simulink model "DriveSystemControl"  (R2025b)
settings: Solver=FixedStepAuto  StartTime=0.0  StopTime=Inf  FixedStep=0.001  RelTol=1e-3
PostLoadFcn:
  | if any(exist('dsrtsu_mdlpostloadfcn', 'file') ~= 0), dsrtsu_mdlpostloadfcn('Execute', bdroot); end
InitFcn:
  | , if any(exist('rtifpga_mdlclblib', 'file') ~= 0), rtifpga_mdlclblib('Init', bdroot); end,
  | , if any(exist('dsmpb_private', 'file') ~= 0), dsmpb_private('dsmpb_mdlclblib', 'Init', bdroot); end,
libraries: dsmpblib x2
(part 8 of 11)

== system DriveSystemControl/Bus Configuration (1) - In/Manipulation/gitam Controller CAN File 08082024/WIP/CANChannel/PDUs/TCU03/sigSupervisorFault/Feature Switch ==
  Const_sigSupervisorFault Countdown Start Value : Constant  Value=0  OutDataTypeStr=uint32
  Const_sigSupervisorFault Feature Switch : Constant  Value=0  OutDataTypeStr=uint32
  _Feature Switch_ : BusCreator  Inputs=2
  Feature Switch : Outport
  wires:
  _Feature Switch_/1 -> Feature Switch/1  "Feature Switch"
  Const_sigSupervisorFault Countdown Start Value/1 -> _Feature Switch_/1  "sigSupervisorFault Countdown Start Value"
  Const_sigSupervisorFault Feature Switch/1 -> _Feature Switch_/2  "sigSupervisorFault Feature Switch"

== system DriveSystemControl/Bus Configuration (1) - In/Manipulation/gitam Controller CAN File 08082024/WIP/CANChannel/PDUs/TCU03/sigSupervisorFault/ISignal Overwrite Value ==
  Const_sigSupervisorFault Overwrite Value : Constant  Value=0  OutDataTypeStr=uint8
  _ISignal Overwrite Value_ : BusCreator  Inputs=1
  ISignal Overwrite Value : Outport
  wires:
  _ISignal Overwrite Value_/1 -> ISignal Overwrite Value/1  "ISignal Overwrite Value"
  Const_sigSupervisorFault Overwrite Value/1 -> _ISignal Overwrite Value_/1  "sigSupervisorFault Overwrite Value"

== system DriveSystemControl/Bus Configuration (1) - In/Manipulation/gitam Controller CAN File 08082024/WIP/CANChannel/PDUs/TCU03/sigThrottlewiperHigh/Feature Switch ==
  Const_sigThrottlewiperHigh Countdown Start Value : Constant  Value=0  OutDataTypeStr=uint32
  Const_sigThrottlewiperHigh Feature Switch : Constant  Value=0  OutDataTypeStr=uint32
  _Feature Switch_ : BusCreator  Inputs=2
  Feature Switch : Outport
  wires:
  _Feature Switch_/1 -> Feature Switch/1  "Feature Switch"
  Const_sigThrottlewiperHigh Countdown Start Value/1 -> _Feature Switch_/1  "sigThrottlewiperHigh Countdown Start Value"
  Const_sigThrottlewiperHigh Feature Switch/1 -> _Feature Switch_/2  "sigThrottlewiperHigh Feature Switch"

== system DriveSystemControl/Bus Configuration (1) - In/Manipulation/gitam Controller CAN File 08082024/WIP/CANChannel/PDUs/TCU03/sigThrottlewiperHigh/ISignal Overwrite Value ==
  Const_sigThrottlewiperHigh Overwrite Value : Constant  Value=0  OutDataTypeStr=uint8
  _ISignal Overwrite Value_ : BusCreator  Inputs=1
  ISignal Overwrite Value : Outport
  wires:
  _ISignal Overwrite Value_/1 -> ISignal Overwrite Value/1  "ISignal Overwrite Value"
  Const_sigThrottlewiperHigh Overwrite Value/1 -> _ISignal Overwrite Value_/1  "sigThrottlewiperHigh Overwrite Value"

== system DriveSystemControl/Bus Configuration (1) - In/Manipulation/gitam Controller CAN File 08082024/WIP/CANChannel/PDUs/TCU03/sigThrottlewiperLow/Feature Switch ==
  Const_sigThrottlewiperLow Countdown Start Value : Constant  Value=0  OutDataTypeStr=uint32
  Const_sigThrottlewiperLow Feature Switch : Constant  Value=0  OutDataTypeStr=uint32
  _Feature Switch_ : BusCreator  Inputs=2
  Feature Switch : Outport
  wires:
  _Feature Switch_/1 -> Feature Switch/1  "Feature Switch"
  Const_sigThrottlewiperLow Countdown Start Value/1 -> _Feature Switch_/1  "sigThrottlewiperLow Countdown Start Value"
  Const_sigThrottlewiperLow Feature Switch/1 -> _Feature Switch_/2  "sigThrottlewiperLow Feature Switch"

== system DriveSystemControl/Bus Configuration (1) - In/Manipulation/gitam Controller CAN File 08082024/WIP/CANChannel/PDUs/TCU03/sigThrottlewiperLow/ISignal Overwrite Value ==
  Const_sigThrottlewiperLow Overwrite Value : Constant  Value=0  OutDataTypeStr=uint8
  _ISignal Overwrite Value_ : BusCreator  Inputs=1
  ISignal Overwrite Value : Outport
  wires:
  _ISignal Overwrite Value_/1 -> ISignal Overwrite Value/1  "ISignal Overwrite Value"
  Const_sigThrottlewiperLow Overwrite Value/1 -> _ISignal Overwrite Value_/1  "sigThrottlewiperLow Overwrite Value"

== system DriveSystemControl/Bus Configuration (1) - In/Manipulation/gitam Controller CAN File 08082024/WIP/CANChannel/PDUs/TCU03/sigVCLRunTimeError/Feature Switch ==
  Const_sigVCLRunTimeError Countdown Start Value : Constant  Value=0  OutDataTypeStr=uint32
  Const_sigVCLRunTimeError Feature Switch : Constant  Value=0  OutDataTypeStr=uint32
  _Feature Switch_ : BusCreator  Inputs=2
  Feature Switch : Outport
  wires:
  _Feature Switch_/1 -> Feature Switch/1  "Feature Switch"
  Const_sigVCLRunTimeError Countdown Start Value/1 -> _Feature Switch_/1  "sigVCLRunTimeError Countdown Start Value"
  Const_sigVCLRunTimeError Feature Switch/1 -> _Feature Switch_/2  "sigVCLRunTimeError Feature Switch"

== system DriveSystemControl/Bus Configuration (1) - In/Manipulation/gitam Controller CAN File 08082024/WIP/CANChannel/PDUs/TCU03/sigVCLRunTimeError/ISignal Overwrite Value ==
  Const_sigVCLRunTimeError Overwrite Value : Constant  Value=0  OutDataTypeStr=uint8
  _ISignal Overwrite Value_ : BusCreator  Inputs=1
  ISignal Overwrite Value : Outport
  wires:
  _ISignal Overwrite Value_/1 -> ISignal Overwrite Value/1  "ISignal Overwrite Value"
  Const_sigVCLRunTimeError Overwrite Value/1 -> _ISignal Overwrite Value_/1  "sigVCLRunTimeError Overwrite Value"

== system DriveSystemControl/Bus Configuration (1) - In/Manipulation/gitam Controller CAN File 08082024/WIP/CANChannel/PDUs/TCU04/sigMCU5_DriveMode/Feature Switch ==
  Const_sigMCU5_DriveMode Countdown Start Value : Constant  Value=0  OutDataTypeStr=uint32
  Const_sigMCU5_DriveMode Feature Switch : Constant  Value=0  OutDataTypeStr=uint32
  _Feature Switch_ : BusCreator  Inputs=2
  Feature Switch : Outport
  wires:
  _Feature Switch_/1 -> Feature Switch/1  "Feature Switch"
  Const_sigMCU5_DriveMode Countdown Start Value/1 -> _Feature Switch_/1  "sigMCU5_DriveMode Countdown Start Value"
  Const_sigMCU5_DriveMode Feature Switch/1 -> _Feature Switch_/2  "sigMCU5_DriveMode Feature Switch"

== system DriveSystemControl/Bus Configuration (1) - In/Manipulation/gitam Controller CAN File 08082024/WIP/CANChannel/PDUs/TCU04/sigMCU5_DriveMode/ISignal Overwrite Value ==
  Const_sigMCU5_DriveMode Overwrite Value : Constant  Value=0  OutDataTypeStr=uint8
  _ISignal Overwrite Value_ : BusCreator  Inputs=1
  ISignal Overwrite Value : Outport
  wires:
  _ISignal Overwrite Value_/1 -> ISignal Overwrite Value/1  "ISignal Overwrite Value"
  Const_sigMCU5_DriveMode Overwrite Value/1 -> _ISignal Overwrite Value_/1  "sigMCU5_DriveMode Overwrite Value"

== system DriveSystemControl/Bus Configuration (1) - In/Manipulation/gitam Controller CAN File 08082024/WIP/CANChannel/PDUs/TCU04/sigMCU5_Efficiency/Feature Switch ==
  Const_sigMCU5_Efficiency Countdown Start Value : Constant  Value=0  OutDataTypeStr=uint32
  Const_sigMCU5_Efficiency Feature Switch : Constant  Value=0  OutDataTypeStr=uint32
  _Feature Switch_ : BusCreator  Inputs=2
  Feature Switch : Outport
  wires:
  _Feature Switch_/1 -> Feature Switch/1  "Feature Switch"
  Const_sigMCU5_Efficiency Countdown Start Value/1 -> _Feature Switch_/1  "sigMCU5_Efficiency Countdown Start Value"
  Const_sigMCU5_Efficiency Feature Switch/1 -> _Feature Switch_/2  "sigMCU5_Efficiency Feature Switch"

== system DriveSystemControl/Bus Configuration (1) - In/Manipulation/gitam Controller CAN File 08082024/WIP/CANChannel/PDUs/TCU04/sigMCU5_Efficiency/ISignal Overwrite Value ==
  Const_sigMCU5_Efficiency Overwrite Value : Constant  Value=0  OutDataTypeStr=uint8
  _ISignal Overwrite Value_ : BusCreator  Inputs=1
  ISignal Overwrite Value : Outport
  wires:
  _ISignal Overwrite Value_/1 -> ISignal Overwrite Value/1  "ISignal Overwrite Value"
  Const_sigMCU5_Efficiency Overwrite Value/1 -> _ISignal Overwrite Value_/1  "sigMCU5_Efficiency Overwrite Value"

== system DriveSystemControl/Bus Configuration (1) - In/Manipulation/gitam Controller CAN File 08082024/WIP/CANChannel/PDUs/TCU04/sigMCU5_Hillhold/Feature Switch ==
  Const_sigMCU5_Hillhold Countdown Start Value : Constant  Value=0  OutDataTypeStr=uint32
  Const_sigMCU5_Hillhold Feature Switch : Constant  Value=0  OutDataTypeStr=uint32
  _Feature Switch_ : BusCreator  Inputs=2
  Feature Switch : Outport
  wires:
  _Feature Switch_/1 -> Feature Switch/1  "Feature Switch"
  Const_sigMCU5_Hillhold Countdown Start Value/1 -> _Feature Switch_/1  "sigMCU5_Hillhold Countdown Start Value"
  Const_sigMCU5_Hillhold Feature Switch/1 -> _Feature Switch_/2  "sigMCU5_Hillhold Feature Switch"

== system DriveSystemControl/Bus Configuration (1) - In/Manipulation/gitam Controller CAN File 08082024/WIP/CANChannel/PDUs/TCU04/sigMCU5_Hillhold/ISignal Overwrite Value ==
  Const_sigMCU5_Hillhold Overwrite Value : Constant  Value=0  OutDataTypeStr=uint8
  _ISignal Overwrite Value_ : BusCreator  Inputs=1
  ISignal Overwrite Value : Outport
  wires:
  _ISignal Overwrite Value_/1 -> ISignal Overwrite Value/1  "ISignal Overwrite Value"
  Const_sigMCU5_Hillhold Overwrite Value/1 -> _ISignal Overwrite Value_/1  "sigMCU5_Hillhold Overwrite Value"

== system DriveSystemControl/Bus Configuration (1) - In/Manipulation/gitam Controller CAN File 08082024/WIP/CANChannel/PDUs/TCU04/sigMCU5_RegenFlag/Feature Switch ==
  Const_sigMCU5_RegenFlag Countdown Start Value : Constant  Value=0  OutDataTypeStr=uint32
  Const_sigMCU5_RegenFlag Feature Switch : Constant  Value=0  OutDataTypeStr=uint32
  _Feature Switch_ : BusCreator  Inputs=2
  Feature Switch : Outport
  wires:
  _Feature Switch_/1 -> Feature Switch/1  "Feature Switch"
  Const_sigMCU5_RegenFlag Countdown Start Value/1 -> _Feature Switch_/1  "sigMCU5_RegenFlag Countdown Start Value"
  Const_sigMCU5_RegenFlag Feature Switch/1 -> _Feature Switch_/2  "sigMCU5_RegenFlag Feature Switch"

== system DriveSystemControl/Bus Configuration (1) - In/Manipulation/gitam Controller CAN File 08082024/WIP/CANChannel/PDUs/TCU04/sigMCU5_RegenFlag/ISignal Overwrite Value ==
  Const_sigMCU5_RegenFlag Overwrite Value : Constant  Value=0  OutDataTypeStr=uint8
  _ISignal Overwrite Value_ : BusCreator  Inputs=1
  ISignal Overwrite Value : Outport
  wires:
  _ISignal Overwrite Value_/1 -> ISignal Overwrite Value/1  "ISignal Overwrite Value"
  Const_sigMCU5_RegenFlag Overwrite Value/1 -> _ISignal Overwrite Value_/1  "sigMCU5_RegenFlag Overwrite Value"

== system DriveSystemControl/Bus Configuration (1) - In/Manipulation/gitam Controller CAN File 08082024/WIP/CANChannel/PDUs/TCU04/sigMCU5_Speed/Feature Switch ==
  Const_sigMCU5_Speed Countdown Start Value : Constant  Value=0  OutDataTypeStr=uint32
  Const_sigMCU5_Speed Feature Switch : Constant  Value=0  OutDataTypeStr=uint32
  _Feature Switch_ : BusCreator  Inputs=2
  Feature Switch : Outport
  wires:
  _Feature Switch_/1 -> Feature Switch/1  "Feature Switch"
  Const_sigMCU5_Speed Countdown Start Value/1 -> _Feature Switch_/1  "sigMCU5_Speed Countdown Start Value"
  Const_sigMCU5_Speed Feature Switch/1 -> _Feature Switch_/2  "sigMCU5_Speed Feature Switch"

== system DriveSystemControl/Bus Configuration (1) - In/Manipulation/gitam Controller CAN File 08082024/WIP/CANChannel/PDUs/TCU04/sigMCU5_Speed/ISignal Overwrite Value ==
  Const_sigMCU5_Speed Overwrite Value : Constant  Value=0  OutDataTypeStr=uint8
  _ISignal Overwrite Value_ : BusCreator  Inputs=1
  ISignal Overwrite Value : Outport
  wires:
  _ISignal Overwrite Value_/1 -> ISignal Overwrite Value/1  "ISignal Overwrite Value"
  Const_sigMCU5_Speed Overwrite Value/1 -> _ISignal Overwrite Value_/1  "sigMCU5_Speed Overwrite Value"

== system DriveSystemControl/Bus Configuration (1) - In/Manipulation/gitam Controller CAN File 08082024/WIP/CANChannel/PDUs/TCU05/sigMCU6_Odometer/Feature Switch ==
  Const_sigMCU6_Odometer Countdown Start Value : Constant  Value=0  OutDataTypeStr=uint32
  Const_sigMCU6_Odometer Feature Switch : Constant  Value=0  OutDataTypeStr=uint32
  _Feature Switch_ : BusCreator  Inputs=2
  Feature Switch : Outport
  wires:
  _Feature Switch_/1 -> Feature Switch/1  "Feature Switch"
  Const_sigMCU6_Odometer Countdown Start Value/1 -> _Feature Switch_/1  "sigMCU6_Odometer Countdown Start Value"
  Const_sigMCU6_Odometer Feature Switch/1 -> _Feature Switch_/2  "sigMCU6_Odometer Feature Switch"

== system DriveSystemControl/Bus Configuration (1) - In/Manipulation/gitam Controller CAN File 08082024/WIP/CANChannel/PDUs/TCU05/sigMCU6_Odometer/ISignal Overwrite Value ==
  Const_sigMCU6_Odometer Overwrite Value : Constant  Value=0  OutDataTypeStr=double
  _ISignal Overwrite Value_ : BusCreator  Inputs=1
  ISignal Overwrite Value : Outport
  wires:
  _ISignal Overwrite Value_/1 -> ISignal Overwrite Value/1  "ISignal Overwrite Value"
  Const_sigMCU6_Odometer Overwrite Value/1 -> _ISignal Overwrite Value_/1  "sigMCU6_Odometer Overwrite Value"

== system DriveSystemControl/Bus Configuration (1) - In/Simulated ECUs/gitam Controller CAN File 08082024/BMS/TX/PDUs/BMS01/sigBatteryMalfunctionLight/ISignal Value ==
  Const_sigBatteryMalfunctionLight Value : Constant  Value=0  OutDataTypeStr=uint8
  _ISignal Value_ : BusCreator  Inputs=1
  ISignal Value : Outport
  wires:
  _ISignal Value_/1 -> ISignal Value/1  "ISignal Value"
  Const_sigBatteryMalfunctionLight Value/1 -> _ISignal Value_/1  "sigBatteryMalfunctionLight Value"

== system DriveSystemControl/Bus Configuration (1) - In/Simulated ECUs/gitam Controller CAN File 08082024/BMS/TX/PDUs/BMS01/sigKeyOnIndicator/ISignal Value ==
  Const_sigKeyOnIndicator Value : Constant  Value=0  OutDataTypeStr=uint8
  _ISignal Value_ : BusCreator  Inputs=1
  ISignal Value : Outport
  wires:
  _ISignal Value_/1 -> ISignal Value/1  "ISignal Value"
  Const_sigKeyOnIndicator Value/1 -> _ISignal Value_/1  "sigKeyOnIndicator Value"

== system DriveSystemControl/Bus Configuration (1) - In/Simulated ECUs/gitam Controller CAN File 08082024/BMS/TX/PDUs/BMS01/sigStateOfCharge/ISignal Value ==
  Const_sigStateOfCharge Value : Constant  Value=0  OutDataTypeStr=uint8
  _ISignal Value_ : BusCreator  Inputs=1
  ISignal Value : Outport
  wires:
  _ISignal Value_/1 -> ISignal Value/1  "ISignal Value"
  Const_sigStateOfCharge Value/1 -> _ISignal Value_/1  "sigStateOfCharge Value"

== system DriveSystemControl/Bus Configuration (1) - In/Simulated ECUs/gitam Controller CAN File 08082024/BMS/TX/PDUs/BMS02/sigBatteryCurrent/ISignal Value ==
  Const_sigBatteryCurrent Value : Constant  Value=0  OutDataTypeStr=double
  _ISignal Value_ : BusCreator  Inputs=1
  ISignal Value : Outport
  wires:
  _ISignal Value_/1 -> ISignal Value/1  "ISignal Value"
  Const_sigBatteryCurrent Value/1 -> _ISignal Value_/1  "sigBatteryCurrent Value"

== system DriveSystemControl/Bus Configuration (1) - In/Simulated ECUs/gitam Controller CAN File 08082024/BMS/TX/PDUs/BMS02/sigDriveCurrentLimit/ISignal Value ==
  Const_sigDriveCurrentLimit Value : Constant  Value=0  OutDataTypeStr=uint8
  _ISignal Value_ : BusCreator  Inputs=1
  ISignal Value : Outport
  wires:
  _ISignal Value_/1 -> ISignal Value/1  "ISignal Value"
  Const_sigDriveCurrentLimit Value/1 -> _ISignal Value_/1  "sigDriveCurrentLimit Value"

== system DriveSystemControl/Bus Configuration (1) - In/Simulated ECUs/gitam Controller CAN File 08082024/BMS/TX/PDUs/BMS02/sigRegenCurrentLimit/ISignal Value ==
  Const_sigRegenCurrentLimit Value : Constant  Value=0  OutDataTypeStr=uint8
  _ISignal Value_ : BusCreator  Inputs=1
  ISignal Value : Outport
  wires:
  _ISignal Value_/1 -> ISignal Value/1  "ISignal Value"
  Const_sigRegenCurrentLimit Value/1 -> _ISignal Value_/1  "sigRegenCurrentLimit Value"

== system DriveSystemControl/Bus Configuration (1) - In/Simulated ECUs/gitam Controller CAN File 08082024/BMS/TX/PDUs/BMS02/sigVehicleModeRequest/ISignal Value ==
  Const_sigVehicleModeRequest Value : Constant  Value=0  OutDataTypeStr=uint8
  _ISignal Value_ : BusCreator  Inputs=1
  ISignal Value : Outport
  wires:
  _ISignal Value_/1 -> ISignal Value/1  "ISignal Value"
  Const_sigVehicleModeRequest Value/1 -> _ISignal Value_/1  "sigVehicleModeRequest Value"

== system DriveSystemControl/Bus Configuration (1) - In/Simulated ECUs/gitam Controller CAN File 08082024/TCU/TX/PDUs/MainController/CCU_heartBeat/ISignal Value ==
  Const_CCU_heartBeat Value : Constant  Value=0  OutDataTypeStr=uint8
  _ISignal Value_ : BusCreator  Inputs=1
  ISignal Value : Outport
  wires:
  _ISignal Value_/1 -> ISignal Value/1  "ISignal Value"
  Const_CCU_heartBeat Value/1 -> _ISignal Value_/1  "CCU_heartBeat Value"

== system DriveSystemControl/Bus Configuration (1) - In/Simulated ECUs/gitam Controller CAN File 08082024/TCU/TX/PDUs/MainController/notUsed/ISignal Value ==
  Const_notUsed Value : Constant  Value=0  OutDataTypeStr=uint8
  _ISignal Value_ : BusCreator  Inputs=1
  ISignal Value : Outport
  wires:
  _ISignal Value_/1 -> ISignal Value/1  "ISignal Value"
  Const_notUsed Value/1 -> _ISignal Value_/1  "notUsed Value"

== system DriveSystemControl/Bus Configuration (1) - In/Simulated ECUs/gitam Controller CAN File 08082024/TCU/TX/PDUs/MainController/setAutoParkBreak/ISignal Value ==
  Const_setAutoParkBreak Value : Constant  Value=0  OutDataTypeStr=uint8
  _ISignal Value_ : BusCreator  Inputs=1
  ISignal Value : Outport
  wires:
  _ISignal Value_/1 -> ISignal Value/1  "ISignal Value"
  Const_setAutoParkBreak Value/1 -> _ISignal Value_/1  "setAutoParkBreak Value"

== system DriveSystemControl/Bus Configuration (1) - In/Simulated ECUs/gitam Controller CAN File 08082024/TCU/TX/PDUs/MainController/setBreake/ISignal Value ==
  Const_setBreake Value : Constant  Value=0  OutDataTypeStr=uint8
  _ISignal Value_ : BusCreator  Inputs=1
  ISignal Value : Outport
  wires:
  _ISignal Value_/1 -> ISignal Value/1  "ISignal Value"
  Const_setBreake Value/1 -> _ISignal Value_/1  "setBreake Value"

== system DriveSystemControl/Bus Configuration (1) - In/Simulated ECUs/gitam Controller CAN File 08082024/TCU/TX/PDUs/MainController/setDirection/ISignal Value ==
  Const_setDirection Value : Constant  Value=0  OutDataTypeStr=uint8
  _ISignal Value_ : BusCreator  Inputs=1
  ISignal Value : Outport
  wires:
  _ISignal Value_/1 -> ISignal Value/1  "ISignal Value"
  Const_setDirection Value/1 -> _ISignal Value_/1  "setDirection Value"

== system DriveSystemControl/Bus Configuration (1) - In/Simulated ECUs/gitam Controller CAN File 08082024/TCU/TX/PDUs/MainController/setDriveMode/ISignal Value ==
  Const_setDriveMode Value : Constant  Value=0  OutDataTypeStr=uint8
  _ISignal Value_ : BusCreator  Inputs=1
  ISignal Value : Outport
  wires:
  _ISignal Value_/1 -> ISignal Value/1  "ISignal Value"
  Const_setDriveMode Value/1 -> _ISignal Value_/1  "setDriveMode Value"

== system DriveSystemControl/Bus Configuration (1) - In/Simulated ECUs/gitam Controller CAN File 08082024/TCU/TX/PDUs/MainController/setVelocity/ISignal Value ==
  Const_setVelocity Value : Constant  Value=127  OutDataTypeStr=uint8
  _ISignal Value_ : BusCreator  Inputs=1
  ISignal Value : Outport
  wires:
  _ISignal Value_/1 -> ISignal Value/1  "ISignal Value"
  Const_setVelocity Value/1 -> _ISignal Value_/1  "setVelocity Value"

== system DriveSystemControl/Bus Configuration (1) - In/Simulated ECUs/gitam Controller CAN File 08082024/TCU/TX/PDUs/MainController/steeringPower/ISignal Value ==
  Const_steeringPower Value : Constant  Value=0  OutDataTypeStr=uint8
  _ISignal Value_ : BusCreator  Inputs=1
  ISignal Value : Outport
  wires:
  _ISignal Value_/1 -> ISignal Value/1  "ISignal Value"
  Const_steeringPower Value/1 -> _ISignal Value_/1  "steeringPower Value"

== system DriveSystemControl/Bus Configuration (1) - In/Simulated ECUs/gitam Controller CAN File 08082024/TCU/TX/PDUs/TCU01/sigBrake/ISignal Value ==
  Const_sigBrake Value : Constant  Value=0  OutDataTypeStr=uint8
  _ISignal Value_ : BusCreator  Inputs=1
  ISignal Value : Outport
  wires:
  _ISignal Value_/1 -> ISignal Value/1  "ISignal Value"
  Const_sigBrake Value/1 -> _ISignal Value_/1  "sigBrake Value"

== system DriveSystemControl/Bus Configuration (1) - In/Simulated ECUs/gitam Controller CAN File 08082024/TCU/TX/PDUs/TCU01/sigControllerTemperature/ISignal Value ==
  Const_sigControllerTemperature Value : Constant  Value=0  OutDataTypeStr=int8
  _ISignal Value_ : BusCreator  Inputs=1
  ISignal Value : Outport
  wires:
  _ISignal Value_/1 -> ISignal Value/1  "ISignal Value"
  Const_sigControllerTemperature Value/1 -> _ISignal Value_/1  "sigControllerTemperature Value"

== system DriveSystemControl/Bus Configuration (1) - In/Simulated ECUs/gitam Controller CAN File 08082024/TCU/TX/PDUs/TCU01/sigDriveMode/ISignal Value ==
  Const_sigDriveMode Value : Constant  Value=0  OutDataTypeStr=uint8
  _ISignal Value_ : BusCreator  Inputs=1
  ISignal Value : Outport
  wires:
  _ISignal Value_/1 -> ISignal Value/1  "ISignal Value"
  Const_sigDriveMode Value/1 -> _ISignal Value_/1  "sigDriveMode Value"

== system DriveSystemControl/Bus Configuration (1) - In/Simulated ECUs/gitam Controller CAN File 08082024/TCU/TX/PDUs/TCU01/sigMotorTemperature/ISignal Value ==
  Const_sigMotorTemperature Value : Constant  Value=-50  OutDataTypeStr=int16
  _ISignal Value_ : BusCreator  Inputs=1
  ISignal Value : Outport
  wires:
  _ISignal Value_/1 -> ISignal Value/1  "ISignal Value"
  Const_sigMotorTemperature Value/1 -> _ISignal Value_/1  "sigMotorTemperature Value"

== system DriveSystemControl/Bus Configuration (1) - In/Simulated ECUs/gitam Controller CAN File 08082024/TCU/TX/PDUs/TCU01/sigRMSCurrent/ISignal Value ==
  Const_sigRMSCurrent Value : Constant  Value=0  OutDataTypeStr=double
  _ISignal Value_ : BusCreator  Inputs=1
  ISignal Value : Outport
  wires:
  _ISignal Value_/1 -> ISignal Value/1  "ISignal Value"
  Const_sigRMSCurrent Value/1 -> _ISignal Value_/1  "sigRMSCurrent Value"

== system DriveSystemControl/Bus Configuration (1) - In/Simulated ECUs/gitam Controller CAN File 08082024/TCU/TX/PDUs/TCU01/sigSpeed/ISignal Value ==
  Const_sigSpeed Value : Constant  Value=0  OutDataTypeStr=uint8
  _ISignal Value_ : BusCreator  Inputs=1
  ISignal Value : Outport
  wires:
  _ISignal Value_/1 -> ISignal Value/1  "ISignal Value"
  Const_sigSpeed Value/1 -> _ISignal Value_/1  "sigSpeed Value"

== system DriveSystemControl/Bus Configuration (1) - In/Simulated ECUs/gitam Controller CAN File 08082024/TCU/TX/PDUs/TCU01/sigThrottle/ISignal Value ==
  Const_sigThrottle Value : Constant  Value=0  OutDataTypeStr=uint8
  _ISignal Value_ : BusCreator  Inputs=1
  ISignal Value : Outport
  wires:
  _ISignal Value_/1 -> ISignal Value/1  "ISignal Value"
  Const_sigThrottle Value/1 -> _ISignal Value_/1  "sigThrottle Value"

== system DriveSystemControl/Bus Configuration (1) - In/Simulated ECUs/gitam Controller CAN File 08082024/TCU/TX/PDUs/TCU02/sigCapacitorVoltage/ISignal Value ==
  Const_sigCapacitorVoltage Value : Constant  Value=0  OutDataTypeStr=double
  _ISignal Value_ : BusCreator  Inputs=1
  ISignal Value : Outport
  wires:
  _ISignal Value_/1 -> ISignal Value/1  "ISignal Value"
  Const_sigCapacitorVoltage Value/1 -> _ISignal Value_/1  "sigCapacitorVoltage Value"

== system DriveSystemControl/Bus Configuration (1) - In/Simulated ECUs/gitam Controller CAN File 08082024/TCU/TX/PDUs/TCU02/sigMotorRPM/ISignal Value ==
  Const_sigMotorRPM Value : Constant  Value=0  OutDataTypeStr=int16
  _ISignal Value_ : BusCreator  Inputs=1
  ISignal Value : Outport
  wires:
  _ISignal Value_/1 -> ISignal Value/1  "ISignal Value"
  Const_sigMotorRPM Value/1 -> _ISignal Value_/1  "sigMotorRPM Value"

== system DriveSystemControl/Bus Configuration (1) - In/Simulated ECUs/gitam Controller CAN File 08082024/TCU/TX/PDUs/TCU02/sigOdometer/ISignal Value ==
  Const_sigOdometer Value : Constant  Value=0  OutDataTypeStr=double
  _ISignal Value_ : BusCreator  Inputs=1
  ISignal Value : Outport
  wires:
  _ISignal Value_/1 -> ISignal Value/1  "ISignal Value"
  Const_sigOdometer Value/1 -> _ISignal Value_/1  "sigOdometer Value"

== system DriveSystemControl/Bus Configuration (1) - In/Simulated ECUs/gitam Controller CAN File 08082024/TCU/TX/PDUs/TCU03/Controller_CompleteFaults/ISignal Value ==
  Const_Controller_CompleteFaults Value : Constant  Value=0  OutDataTypeStr=uint8
  _ISignal Value_ : BusCreator  Inputs=1
  ISignal Value : Outport
  wires:
  _ISignal Value_/1 -> ISignal Value/1  "ISignal Value"
  Const_Controller_CompleteFaults Value/1 -> _ISignal Value_/1  "Controller_CompleteFaults Value"

== system DriveSystemControl/Bus Configuration (1) - In/Simulated ECUs/gitam Controller CAN File 08082024/TCU/TX/PDUs/TCU03/sig5VSupplyFailure/ISignal Value ==
  Const_sig5VSupplyFailure Value : Constant  Value=0  OutDataTypeStr=uint8
  _ISignal Value_ : BusCreator  Inputs=1
  ISignal Value : Outport
  wires:
  _ISignal Value_/1 -> ISignal Value/1  "ISignal Value"
  Const_sig5VSupplyFailure Value/1 -> _ISignal Value_/1  "sig5VSupplyFailure Value"

== system DriveSystemControl/Bus Configuration (1) - In/Simulated ECUs/gitam Controller CAN File 08082024/TCU/TX/PDUs/TCU03/sigBPosOvervoltageCutback/ISignal Value ==
  Const_sigBPosOvervoltageCutback Value : Constant  Value=0  OutDataTypeStr=uint8
  _ISignal Value_ : BusCreator  Inputs=1
  ISignal Value : Outport
  wires:
  _ISignal Value_/1 -> ISignal Value/1  "ISignal Value"
  Const_sigBPosOvervoltageCutback Value/1 -> _ISignal Value_/1  "sigBPosOvervoltageCutback Value"

== system DriveSystemControl/Bus Configuration (1) - In/Simulated ECUs/gitam Controller CAN File 08082024/TCU/TX/PDUs/TCU03/sigBPosUndervoltageCutback/ISignal Value ==
  Const_sigBPosUndervoltageCutback Value : Constant  Value=0  OutDataTypeStr=uint8
  _ISignal Value_ : BusCreator  Inputs=1
  ISignal Value : Outport
  wires:
  _ISignal Value_/1 -> ISignal Value/1  "ISignal Value"
  Const_sigBPosUndervoltageCutback Value/1 -> _ISignal Value_/1  "sigBPosUndervoltageCutback Value"

== system DriveSystemControl/Bus Configuration (1) - In/Simulated ECUs/gitam Controller CAN File 08082024/TCU/TX/PDUs/TCU03/sigBadCalibration/ISignal Value ==
  Const_sigBadCalibration Value : Constant  Value=0  OutDataTypeStr=uint8
  _ISignal Value_ : BusCreator  Inputs=1
  ISignal Value : Outport
  wires:
  _ISignal Value_/1 -> ISignal Value/1  "ISignal Value"
  Const_sigBadCalibration Value/1 -> _ISignal Value_/1  "sigBadCalibration Value"

== system DriveSystemControl/Bus Configuration (1) - In/Simulated ECUs/gitam Controller CAN File 08082024/TCU/TX/PDUs/TCU03/sigBrakeWiperHigh/ISignal Value ==
  Const_sigBrakeWiperHigh Value : Constant  Value=0  OutDataTypeStr=uint8
  _ISignal Value_ : BusCreator  Inputs=1
  ISignal Value : Outport
  wires:
  _ISignal Value_/1 -> ISignal Value/1  "ISignal Value"
  Const_sigBrakeWiperHigh Value/1 -> _ISignal Value_/1  "sigBrakeWiperHigh Value"

== system DriveSystemControl/Bus Configuration (1) - In/Simulated ECUs/gitam Controller CAN File 08082024/TCU/TX/PDUs/TCU03/sigBrakeWiperLow/ISignal Value ==
  Const_sigBrakeWiperLow Value : Constant  Value=0  OutDataTypeStr=uint8
  _ISignal Value_ : BusCreator  Inputs=1
  ISignal Value : Outport
  wires:
  _ISignal Value_/1 -> ISignal Value/1  "ISignal Value"
  Const_sigBrakeWiperLow Value/1 -> _ISignal Value_/1  "sigBrakeWiperLow Value"

== system DriveSystemControl/Bus Configuration (1) - In/Simulated ECUs/gitam Controller CAN File 08082024/TCU/TX/PDUs/TCU03/sigCoil2DriverOpenShort/ISignal Value ==
  Const_sigCoil2DriverOpenShort Value : Constant  Value=0  OutDataTypeStr=uint8
  _ISignal Value_ : BusCreator  Inputs=1
  ISignal Value : Outport
  wires:
  _ISignal Value_/1 -> ISignal Value/1  "ISignal Value"
  Const_sigCoil2DriverOpenShort Value/1 -> _ISignal Value_/1  "sigCoil2DriverOpenShort Value"

== system DriveSystemControl/Bus Configuration (1) - In/Simulated ECUs/gitam Controller CAN File 08082024/TCU/TX/PDUs/TCU03/sigCoil3DriverOpenShort/ISignal Value ==
  Const_sigCoil3DriverOpenShort Value : Constant  Value=0  OutDataTypeStr=uint8
  _ISignal Value_ : BusCreator  Inputs=1
  ISignal Value : Outport
  wires:
  _ISignal Value_/1 -> ISignal Value/1  "ISignal Value"
  Const_sigCoil3DriverOpenShort Value/1 -> _ISignal Value_/1  "sigCoil3DriverOpenShort Value"

== system DriveSystemControl/Bus Configuration (1) - In/Simulated ECUs/gitam Controller CAN File 08082024/TCU/TX/PDUs/TCU03/sigCoil4DriverOpenShort/ISignal Value ==
  Const_sigCoil4DriverOpenShort Value : Constant  Value=0  OutDataTypeStr=uint8
  _ISignal Value_ : BusCreator  Inputs=1
  ISignal Value : Outport
  wires:
  _ISignal Value_/1 -> ISignal Value/1  "ISignal Value"
  Const_sigCoil4DriverOpenShort Value/1 -> _ISignal Value_/1  "sigCoil4DriverOpenShort Value"

== system DriveSystemControl/Bus Configuration (1) - In/Simulated ECUs/gitam Controller CAN File 08082024/TCU/TX/PDUs/TCU03/sigControllerCommonFault/ISignal Value ==
  Const_sigControllerCommonFault Value : Constant  Value=0  OutDataTypeStr=uint8
  _ISignal Value_ : BusCreator  Inputs=1
  ISignal Value : Outport
  wires:
  _ISignal Value_/1 -> ISignal Value/1  "ISignal Value"
  Const_sigControllerCommonFault Value/1 -> _ISignal Value_/1  "sigControllerCommonFault Value"

== system DriveSystemControl/Bus Configuration (1) - In/Simulated ECUs/gitam Controller CAN File 08082024/TCU/TX/PDUs/TCU03/sigControllerOverCurrent/ISignal Value ==
  Const_sigControllerOverCurrent Value : Constant  Value=0  OutDataTypeStr=uint8
  _ISignal Value_ : BusCreator  Inputs=1
  ISignal Value : Outport
  wires:
  _ISignal Value_/1 -> ISignal Value/1  "ISignal Value"
  Const_sigControllerOverCurrent Value/1 -> _ISignal Value_/1  "sigControllerOverCurrent Value"

== system DriveSystemControl/Bus Configuration (1) - In/Simulated ECUs/gitam Controller CAN File 08082024/TCU/TX/PDUs/TCU03/sigControllerOvertempCutback/ISignal Value ==
  Const_sigControllerOvertempCutback Value : Constant  Value=0  OutDataTypeStr=uint8
  _ISignal Value_ : BusCreator  Inputs=1
  ISignal Value : Outport
  wires:
  _ISignal Value_/1 -> ISignal Value/1  "ISignal Value"
  Const_sigControllerOvertempCutback Value/1 -> _ISignal Value_/1  "sigControllerOvertempCutback Value"

== system DriveSystemControl/Bus Configuration (1) - In/Simulated ECUs/gitam Controller CAN File 08082024/TCU/TX/PDUs/TCU03/sigControllerSevereOvertemp/ISignal Value ==
  Const_sigControllerSevereOvertemp Value : Constant  Value=0  OutDataTypeStr=uint8
  _ISignal Value_ : BusCreator  Inputs=1
  ISignal Value : Outport
  wires:
  _ISignal Value_/1 -> ISignal Value/1  "ISignal Value"
  Const_sigControllerSevereOvertemp Value/1 -> _ISignal Value_/1  "sigControllerSevereOvertemp Value"

== system DriveSystemControl/Bus Configuration (1) - In/Simulated ECUs/gitam Controller CAN File 08082024/TCU/TX/PDUs/TCU03/sigControllerSevereUndertemp/ISignal Value ==
  Const_sigControllerSevereUndertemp Value : Constant  Value=0  OutDataTypeStr=uint8
  _ISignal Value_ : BusCreator  Inputs=1
  ISignal Value : Outport
  wires:
  _ISignal Value_/1 -> ISignal Value/1  "ISignal Value"
  Const_sigControllerSevereUndertemp Value/1 -> _ISignal Value_/1  "sigControllerSevereUndertemp Value"

== system DriveSystemControl/Bus Configuration (1) - In/Simulated ECUs/gitam Controller CAN File 08082024/TCU/TX/PDUs/TCU03/sigCurrentSensorFault/ISignal Value ==
  Const_sigCurrentSensorFault Value : Constant  Value=0  OutDataTypeStr=uint8
  _ISignal Value_ : BusCreator  Inputs=1
  ISignal Value : Outport
  wires:
  _ISignal Value_/1 -> ISignal Value/1  "ISignal Value"
  Const_sigCurrentSensorFault Value/1 -> _ISignal Value_/1  "sigCurrentSensorFault Value"

== system DriveSystemControl/Bus Configuration (1) - In/Simulated ECUs/gitam Controller CAN File 08082024/TCU/TX/PDUs/TCU03/sigEEPROMFailure/ISignal Value ==
  Const_sigEEPROMFailure Value : Constant  Value=0  OutDataTypeStr=uint8
  _ISignal Value_ : BusCreator  Inputs=1
  ISignal Value : Outport
  wires:
  _ISignal Value_/1 -> ISignal Value/1  "ISignal Value"
  Const_sigEEPROMFailure Value/1 -> _ISignal Value_/1  "sigEEPROMFailure Value"

== system DriveSystemControl/Bus Configuration (1) - In/Simulated ECUs/gitam Controller CAN File 08082024/TCU/TX/PDUs/TCU03/sigHighPedalDisable/ISignal Value ==
  Const_sigHighPedalDisable Value : Constant  Value=0  OutDataTypeStr=uint8
  _ISignal Value_ : BusCreator  Inputs=1
  ISignal Value : Outport
  wires:
  _ISignal Value_/1 -> ISignal Value/1  "ISignal Value"
  Const_sigHighPedalDisable Value/1 -> _ISignal Value_/1  "sigHighPedalDisable Value"

== system DriveSystemControl/Bus Configuration (1) - In/Simulated ECUs/gitam Controller CAN File 08082024/TCU/TX/PDUs/TCU03/sigInsulationResistanceLow/ISignal Value ==
  Const_sigInsulationResistanceLow Value : Constant  Value=0  OutDataTypeStr=uint8
  _ISignal Value_ : BusCreator  Inputs=1
  ISignal Value : Outport
  wires:
  _ISignal Value_/1 -> ISignal Value/1  "ISignal Value"
  Const_sigInsulationResistanceLow Value/1 -> _ISignal Value_/1  "sigInsulationResistanceLow Value"

== system DriveSystemControl/Bus Configuration (1) - In/Simulated ECUs/gitam Controller CAN File 08082024/TCU/TX/PDUs/TCU03/sigMainContactorWelded/ISignal Value ==
  Const_sigMainContactorWelded Value : Constant  Value=0  OutDataTypeStr=uint8
  _ISignal Value_ : BusCreator  Inputs=1
  ISignal Value : Outport
  wires:
  _ISignal Value_/1 -> ISignal Value/1  "ISignal Value"
  Const_sigMainContactorWelded Value/1 -> _ISignal Value_/1  "sigMainContactorWelded Value"

== system DriveSystemControl/Bus Configuration (1) - In/Simulated ECUs/gitam Controller CAN File 08082024/TCU/TX/PDUs/TCU03/sigMainContactordidnotClose/ISignal Value ==
  Const_sigMainContactordidnotClose Value : Constant  Value=0  OutDataTypeStr=uint8
  _ISignal Value_ : BusCreator  Inputs=1
  ISignal Value : Outport
  wires:
  _ISignal Value_/1 -> ISignal Value/1  "ISignal Value"
  Const_sigMainContactordidnotClose Value/1 -> _ISignal Value_/1  "sigMainContactordidnotClose Value"

== system DriveSystemControl/Bus Configuration (1) - In/Simulated ECUs/gitam Controller CAN File 08082024/TCU/TX/PDUs/TCU03/sigMainOpenShort/ISignal Value ==
  Const_sigMainOpenShort Value : Constant  Value=0  OutDataTypeStr=uint8
  _ISignal Value_ : BusCreator  Inputs=1
  ISignal Value : Outport
  wires:
  _ISignal Value_/1 -> ISignal Value/1  "ISignal Value"
  Const_sigMainOpenShort Value/1 -> _ISignal Value_/1  "sigMainOpenShort Value"

== system DriveSystemControl/Bus Configuration (1) - In/Simulated ECUs/gitam Controller CAN File 08082024/TCU/TX/PDUs/TCU03/sigMotorCharacterization/ISignal Value ==
  Const_sigMotorCharacterization Value : Constant  Value=0  OutDataTypeStr=uint8
  _ISignal Value_ : BusCreator  Inputs=1
  ISignal Value : Outport
  wires:
  _ISignal Value_/1 -> ISignal Value/1  "ISignal Value"
  Const_sigMotorCharacterization Value/1 -> _ISignal Value_/1  "sigMotorCharacterization Value"

== system DriveSystemControl/Bus Configuration (1) - In/Simulated ECUs/gitam Controller CAN File 08082024/TCU/TX/PDUs/TCU03/sigMotorPhaseOpen/ISignal Value ==
  Const_sigMotorPhaseOpen Value : Constant  Value=0  OutDataTypeStr=uint8
  _ISignal Value_ : BusCreator  Inputs=1
  ISignal Value : Outport
  wires:
  _ISignal Value_/1 -> ISignal Value/1  "ISignal Value"
  Const_sigMotorPhaseOpen Value/1 -> _ISignal Value_/1  "sigMotorPhaseOpen Value"

== system DriveSystemControl/Bus Configuration (1) - In/Simulated ECUs/gitam Controller CAN File 08082024/TCU/TX/PDUs/TCU03/sigMotorTempHotCutback/ISignal Value ==
  Const_sigMotorTempHotCutback Value : Constant  Value=0  OutDataTypeStr=uint8
  _ISignal Value_ : BusCreator  Inputs=1
  ISignal Value : Outport
  wires:
  _ISignal Value_/1 -> ISignal Value/1  "ISignal Value"
  Const_sigMotorTempHotCutback Value/1 -> _ISignal Value_/1  "sigMotorTempHotCutback Value"

== system DriveSystemControl/Bus Configuration (1) - In/Simulated ECUs/gitam Controller CAN File 08082024/TCU/TX/PDUs/TCU03/sigMotorTempSensorFault/ISignal Value ==
  Const_sigMotorTempSensorFault Value : Constant  Value=0  OutDataTypeStr=uint8
  _ISignal Value_ : BusCreator  Inputs=1
  ISignal Value : Outport
  wires:
  _ISignal Value_/1 -> ISignal Value/1  "ISignal Value"
  Const_sigMotorTempSensorFault Value/1 -> _ISignal Value_/1  "sigMotorTempSensorFault Value"

== system DriveSystemControl/Bus Configuration (1) - In/Simulated ECUs/gitam Controller CAN File 08082024/TCU/TX/PDUs/TCU03/sigOEM_BatterySTOPSignal/ISignal Value ==
  Const_sigOEM_BatterySTOPSignal Value : Constant  Value=0  OutDataTypeStr=uint8
  _ISignal Value_ : BusCreator  Inputs=1
  ISignal Value : Outport
  wires:
  _ISignal Value_/1 -> ISignal Value/1  "ISignal Value"
  Const_sigOEM_BatterySTOPSignal Value/1 -> _ISignal Value_/1  "sigOEM_BatterySTOPSignal Value"

== system DriveSystemControl/Bus Configuration (1) - In/Simulated ECUs/gitam Controller CAN File 08082024/TCU/TX/PDUs/TCU03/sigOEM_NoBatteryCAN/ISignal Value ==
  Const_sigOEM_NoBatteryCAN Value : Constant  Value=0  OutDataTypeStr=uint8
  _ISignal Value_ : BusCreator  Inputs=1
  ISignal Value : Outport
  wires:
  _ISignal Value_/1 -> ISignal Value/1  "ISignal Value"
  Const_sigOEM_NoBatteryCAN Value/1 -> _ISignal Value_/1  "sigOEM_NoBatteryCAN Value"

== system DriveSystemControl/Bus Configuration (1) - In/Simulated ECUs/gitam Controller CAN File 08082024/TCU/TX/PDUs/TCU03/sigOSGeneral/ISignal Value ==
  Const_sigOSGeneral Value : Constant  Value=0  OutDataTypeStr=uint8
  _ISignal Value_ : BusCreator  Inputs=1
  ISignal Value : Outport
  wires:
  _ISignal Value_/1 -> ISignal Value/1  "ISignal Value"
  Const_sigOSGeneral Value/1 -> _ISignal Value_/1  "sigOSGeneral Value"

== system DriveSystemControl/Bus Configuration (1) - In/Simulated ECUs/gitam Controller CAN File 08082024/TCU/TX/PDUs/TCU03/sigPMACCommissioningNeeded/ISignal Value ==
  Const_sigPMACCommissioningNeeded Value : Constant  Value=0  OutDataTypeStr=uint8
  _ISignal Value_ : BusCreator  Inputs=1
  ISignal Value : Outport
  wires:
  _ISignal Value_/1 -> ISignal Value/1  "ISignal Value"
  Const_sigPMACCommissioningNeeded Value/1 -> _ISignal Value_/1  "sigPMACCommissioningNeeded Value"

== system DriveSystemControl/Bus Configuration (1) - In/Simulated ECUs/gitam Controller CAN File 08082024/TCU/TX/PDUs/TCU03/sigParameterChangeFault/ISignal Value ==
  Const_sigParameterChangeFault Value : Constant  Value=0  OutDataTypeStr=uint8
  _ISignal Value_ : BusCreator  Inputs=1
  ISignal Value : Outport
  wires:
  _ISignal Value_/1 -> ISignal Value/1  "ISignal Value"
  Const_sigParameterChangeFault Value/1 -> _ISignal Value_/1  "sigParameterChangeFault Value"

== system DriveSystemControl/Bus Configuration (1) - In/Simulated ECUs/gitam Controller CAN File 08082024/TCU/TX/PDUs/TCU03/sigPhasePWMMismatch/ISignal Value ==
  Const_sigPhasePWMMismatch Value : Constant  Value=0  OutDataTypeStr=uint8
  _ISignal Value_ : BusCreator  Inputs=1
  ISignal Value : Outport
  wires:
  _ISignal Value_/1 -> ISignal Value/1  "ISignal Value"
  Const_sigPhasePWMMismatch Value/1 -> _ISignal Value_/1  "sigPhasePWMMismatch Value"

== system DriveSystemControl/Bus Configuration (1) - In/Simulated ECUs/gitam Controller CAN File 08082024/TCU/TX/PDUs/TCU03/sigPrechargeFailed/ISignal Value ==
  Const_sigPrechargeFailed Value : Constant  Value=0  OutDataTypeStr=uint8
  _ISignal Value_ : BusCreator  Inputs=1
  ISignal Value : Outport
  wires:
  _ISignal Value_/1 -> ISignal Value/1  "ISignal Value"
  Const_sigPrechargeFailed Value/1 -> _ISignal Value_/1  "sigPrechargeFailed Value"

== system DriveSystemControl/Bus Configuration (1) - In/Simulated ECUs/gitam Controller CAN File 08082024/TCU/TX/PDUs/TCU03/sigSevereBPosOvervoltage/ISignal Value ==
  Const_sigSevereBPosOvervoltage Value : Constant  Value=0  OutDataTypeStr=uint8
  _ISignal Value_ : BusCreator  Inputs=1
  ISignal Value : Outport
  wires:
  _ISignal Value_/1 -> ISignal Value/1  "ISignal Value"
  Const_sigSevereBPosOvervoltage Value/1 -> _ISignal Value_/1  "sigSevereBPosOvervoltage Value"

== system DriveSystemControl/Bus Configuration (1) - In/Simulated ECUs/gitam Controller CAN File 08082024/TCU/TX/PDUs/TCU03/sigSevereBPosUndervoltage/ISignal Value ==
  Const_sigSevereBPosUndervoltage Value : Constant  Value=0  OutDataTypeStr=uint8
  _ISignal Value_ : BusCreator  Inputs=1
  ISignal Value : Outport
  wires:
  _ISignal Value_/1 -> ISignal Value/1  "ISignal Value"
  Const_sigSevereBPosUndervoltage Value/1 -> _ISignal Value_/1  "sigSevereBPosUndervoltage Value"

== system DriveSystemControl/Bus Configuration (1) - In/Simulated ECUs/gitam Controller CAN File 08082024/TCU/TX/PDUs/TCU03/sigSevereKSIOvervoltage/ISignal Value ==
  Const_sigSevereKSIOvervoltage Value : Constant  Value=0  OutDataTypeStr=uint8
  _ISignal Value_ : BusCreator  Inputs=1
  ISignal Value : Outport
  wires:
  _ISignal Value_/1 -> ISignal Value/1  "ISignal Value"
  Const_sigSevereKSIOvervoltage Value/1 -> _ISignal Value_/1  "sigSevereKSIOvervoltage Value"

== system DriveSystemControl/Bus Configuration (1) - In/Simulated ECUs/gitam Controller CAN File 08082024/TCU/TX/PDUs/TCU03/sigSevereKSIUndervoltage/ISignal Value ==
  Const_sigSevereKSIUndervoltage Value : Constant  Value=0  OutDataTypeStr=uint8
  _ISignal Value_ : BusCreator  Inputs=1
  ISignal Value : Outport
  wires:
  _ISignal Value_/1 -> ISignal Value/1  "ISignal Value"
  Const_sigSevereKSIUndervoltage Value/1 -> _ISignal Value_/1  "sigSevereKSIUndervoltage Value"

== system DriveSystemControl/Bus Configuration (1) - In/Simulated ECUs/gitam Controller CAN File 08082024/TCU/TX/PDUs/TCU03/sigSinCosMisalignment/ISignal Value ==
  Const_sigSinCosMisalignment Value : Constant  Value=0  OutDataTypeStr=uint8
  _ISignal Value_ : BusCreator  Inputs=1
  ISignal Value : Outport
  wires:
  _ISignal Value_/1 -> ISignal Value/1  "ISignal Value"
  Const_sigSinCosMisalignment Value/1 -> _ISignal Value_/1  "sigSinCosMisalignment Value"

== system DriveSystemControl/Bus Configuration (1) - In/Simulated ECUs/gitam Controller CAN File 08082024/TCU/TX/PDUs/TCU03/sigSinCosSensorFault/ISignal Value ==
  Const_sigSinCosSensorFault Value : Constant  Value=0  OutDataTypeStr=uint8
  _ISignal Value_ : BusCreator  Inputs=1
  ISignal Value : Outport
  wires:
  _ISignal Value_/1 -> ISignal Value/1  "ISignal Value"
  Const_sigSinCosSensorFault Value/1 -> _ISignal Value_/1  "sigSinCosSensorFault Value"

== system DriveSystemControl/Bus Configuration (1) - In/Simulated ECUs/gitam Controller CAN File 08082024/TCU/TX/PDUs/TCU03/sigStallDetected/ISignal Value ==
  Const_sigStallDetected Value : Constant  Value=0  OutDataTypeStr=uint8
  _ISignal Value_ : BusCreator  Inputs=1
  ISignal Value : Outport
  wires:
  _ISignal Value_/1 -> ISignal Value/1  "ISignal Value"
  Const_sigStallDetected Value/1 -> _ISignal Value_/1  "sigStallDetected Value"

== system DriveSystemControl/Bus Configuration (1) - In/Simulated ECUs/gitam Controller CAN File 08082024/TCU/TX/PDUs/TCU03/sigSupervisorFault/ISignal Value ==
  Const_sigSupervisorFault Value : Constant  Value=0  OutDataTypeStr=uint8
  _ISignal Value_ : BusCreator  Inputs=1
  ISignal Value : Outport
  wires:
  _ISignal Value_/1 -> ISignal Value/1  "ISignal Value"
  Const_sigSupervisorFault Value/1 -> _ISignal Value_/1  "sigSupervisorFault Value"

== system DriveSystemControl/Bus Configuration (1) - In/Simulated ECUs/gitam Controller CAN File 08082024/TCU/TX/PDUs/TCU03/sigThrottlewiperHigh/ISignal Value ==
  Const_sigThrottlewiperHigh Value : Constant  Value=0  OutDataTypeStr=uint8
  _ISignal Value_ : BusCreator  Inputs=1
  ISignal Value : Outport
  wires:
  _ISignal Value_/1 -> ISignal Value/1  "ISignal Value"
  Const_sigThrottlewiperHigh Value/1 -> _ISignal Value_/1  "sigThrottlewiperHigh Value"

== system DriveSystemControl/Bus Configuration (1) - In/Simulated ECUs/gitam Controller CAN File 08082024/TCU/TX/PDUs/TCU03/sigThrottlewiperLow/ISignal Value ==
  Const_sigThrottlewiperLow Value : Constant  Value=0  OutDataTypeStr=uint8
  _ISignal Value_ : BusCreator  Inputs=1
  ISignal Value : Outport
  wires:
  _ISignal Value_/1 -> ISignal Value/1  "ISignal Value"
  Const_sigThrottlewiperLow Value/1 -> _ISignal Value_/1  "sigThrottlewiperLow Value"

== system DriveSystemControl/Bus Configuration (1) - In/Simulated ECUs/gitam Controller CAN File 08082024/TCU/TX/PDUs/TCU03/sigVCLRunTimeError/ISignal Value ==
  Const_sigVCLRunTimeError Value : Constant  Value=0  OutDataTypeStr=uint8
  _ISignal Value_ : BusCreator  Inputs=1
  ISignal Value : Outport
  wires:
  _ISignal Value_/1 -> ISignal Value/1  "ISignal Value"
  Const_sigVCLRunTimeError Value/1 -> _ISignal Value_/1  "sigVCLRunTimeError Value"

== system DriveSystemControl/Bus Configuration (1) - In/Simulated ECUs/gitam Controller CAN File 08082024/TCU/TX/PDUs/TCU04/sigMCU5_DriveMode/ISignal Value ==
  Const_sigMCU5_DriveMode Value : Constant  Value=0  OutDataTypeStr=uint8
  _ISignal Value_ : BusCreator  Inputs=1
  ISignal Value : Outport
  wires:
  _ISignal Value_/1 -> ISignal Value/1  "ISignal Value"
  Const_sigMCU5_DriveMode Value/1 -> _ISignal Value_/1  "sigMCU5_DriveMode Value"

== system DriveSystemControl/Bus Configuration (1) - In/Simulated ECUs/gitam Controller CAN File 08082024/TCU/TX/PDUs/TCU04/sigMCU5_Efficiency/ISignal Value ==
  Const_sigMCU5_Efficiency Value : Constant  Value=0  OutDataTypeStr=uint8
  _ISignal Value_ : BusCreator  Inputs=1
  ISignal Value : Outport
  wires:
  _ISignal Value_/1 -> ISignal Value/1  "ISignal Value"
  Const_sigMCU5_Efficiency Value/1 -> _ISignal Value_/1  "sigMCU5_Efficiency Value"

== system DriveSystemControl/Bus Configuration (1) - In/Simulated ECUs/gitam Controller CAN File 08082024/TCU/TX/PDUs/TCU04/sigMCU5_Hillhold/ISignal Value ==
  Const_sigMCU5_Hillhold Value : Constant  Value=0  OutDataTypeStr=uint8
  _ISignal Value_ : BusCreator  Inputs=1
  ISignal Value : Outport
  wires:
  _ISignal Value_/1 -> ISignal Value/1  "ISignal Value"
  Const_sigMCU5_Hillhold Value/1 -> _ISignal Value_/1  "sigMCU5_Hillhold Value"

== system DriveSystemControl/Bus Configuration (1) - In/Simulated ECUs/gitam Controller CAN File 08082024/TCU/TX/PDUs/TCU04/sigMCU5_RegenFlag/ISignal Value ==
  Const_sigMCU5_RegenFlag Value : Constant  Value=0  OutDataTypeStr=uint8
  _ISignal Value_ : BusCreator  Inputs=1
  ISignal Value : Outport
  wires:
  _ISignal Value_/1 -> ISignal Value/1  "ISignal Value"
  Const_sigMCU5_RegenFlag Value/1 -> _ISignal Value_/1  "sigMCU5_RegenFlag Value"

== system DriveSystemControl/Bus Configuration (1) - In/Simulated ECUs/gitam Controller CAN File 08082024/TCU/TX/PDUs/TCU04/sigMCU5_Speed/ISignal Value ==
  Const_sigMCU5_Speed Value : Constant  Value=0  OutDataTypeStr=uint8
  _ISignal Value_ : BusCreator  Inputs=1
  ISignal Value : Outport
  wires:
  _ISignal Value_/1 -> ISignal Value/1  "ISignal Value"
  Const_sigMCU5_Speed Value/1 -> _ISignal Value_/1  "sigMCU5_Speed Value"

== system DriveSystemControl/Bus Configuration (1) - In/Simulated ECUs/gitam Controller CAN File 08082024/TCU/TX/PDUs/TCU05/sigMCU6_Odometer/ISignal Value ==
  Const_sigMCU6_Odometer Value : Constant  Value=0  OutDataTypeStr=double
  _ISignal Value_ : BusCreator  Inputs=1
  ISignal Value : Outport
  wires:
  _ISignal Value_/1 -> ISignal Value/1  "ISignal Value"
  Const_sigMCU6_Odometer Value/1 -> _ISignal Value_/1  "sigMCU6_Odometer Value"

== system DriveSystemControl/Bus Configuration (1) - Out/Manipulation/gitam Controller CAN File 08082024/WIP/CANChannel/PDUs/BMS01/sigBatteryMalfunctionLight/Feature Switch ==
  Feature Switch : Inport
  Term_sigBatteryMalfunctionLight Current Countdown Value : Terminator
  Term_sigBatteryMalfunctionLight Selected Feature : Terminator
  _Feature Switch_ : BusSelector  OutputSignals=sigBatteryMalfunctionLight Current Countdown Value,sigBatteryMalfunctionLight Selected Feature
  wires:
  Feature Switch/1 -> _Feature Switch_/1  "Feature Switch"
  _Feature Switch_/1 -> Term_sigBatteryMalfunctionLight Current Countdown Value/1  "<sigBatteryMalfunctionLight Current Countdown Value>"
  _Feature Switch_/2 -> Term_sigBatteryMalfunctionLight Selected Feature/1  "<sigBatteryMalfunctionLight Selected Feature>"

== system DriveSystemControl/Bus Configuration (1) - Out/Manipulation/gitam Controller CAN File 08082024/WIP/CANChannel/PDUs/BMS01/sigKeyOnIndicator/Feature Switch ==
  Feature Switch : Inport
  Term_sigKeyOnIndicator Current Countdown Value : Terminator
  Term_sigKeyOnIndicator Selected Feature : Terminator
  _Feature Switch_ : BusSelector  OutputSignals=sigKeyOnIndicator Current Countdown Value,sigKeyOnIndicator Selected Feature
  wires:
  Feature Switch/1 -> _Feature Switch_/1  "Feature Switch"
  _Feature Switch_/1 -> Term_sigKeyOnIndicator Current Countdown Value/1  "<sigKeyOnIndicator Current Countdown Value>"
  _Feature Switch_/2 -> Term_sigKeyOnIndicator Selected Feature/1  "<sigKeyOnIndicator Selected Feature>"

== system DriveSystemControl/Bus Configuration (1) - Out/Manipulation/gitam Controller CAN File 08082024/WIP/CANChannel/PDUs/BMS01/sigStateOfCharge/Feature Switch ==
  Feature Switch : Inport
  Term_sigStateOfCharge Current Countdown Value : Terminator
  Term_sigStateOfCharge Selected Feature : Terminator
  _Feature Switch_ : BusSelector  OutputSignals=sigStateOfCharge Current Countdown Value,sigStateOfCharge Selected Feature
  wires:
  Feature Switch/1 -> _Feature Switch_/1  "Feature Switch"
  _Feature Switch_/1 -> Term_sigStateOfCharge Current Countdown Value/1  "<sigStateOfCharge Current Countdown Value>"
  _Feature Switch_/2 -> Term_sigStateOfCharge Selected Feature/1  "<sigStateOfCharge Selected Feature>"
